simulink model "gm_soc_dvbs2_fpga"  (R2025b)
settings: Solver=VariableStepAuto  StartTime=0.0  StopTime=10.0  RelTol=1e-3
InitFcn:
  | soc_dvbs2_init;
undefined symbols (not defined in the file or in its folder): Add, coefficientsLog, coefficientsSqrt1, coefficientsSqrt2, dataBits, Deinterleaver, designMultirateFIR, noisePow, Shift, Short, soc_dvbs2_designFIRFilter, soc_dvbs2_txPacketBits, syncWord, txDataOut, txFiltCoeff, XData
libraries: simulink x304, hdlsllib x265, dspsigops x15, dsphdlfiltering2 x8, hdlmdlgenlib x6, dsphdlsigops2 x5, commseqgen3 x5, dsphdlmathfun2 x3, hwlogicconnlib x2, whdledac x2, commhdlcrc x2, whdlutilities x1
(part 3 of 36)

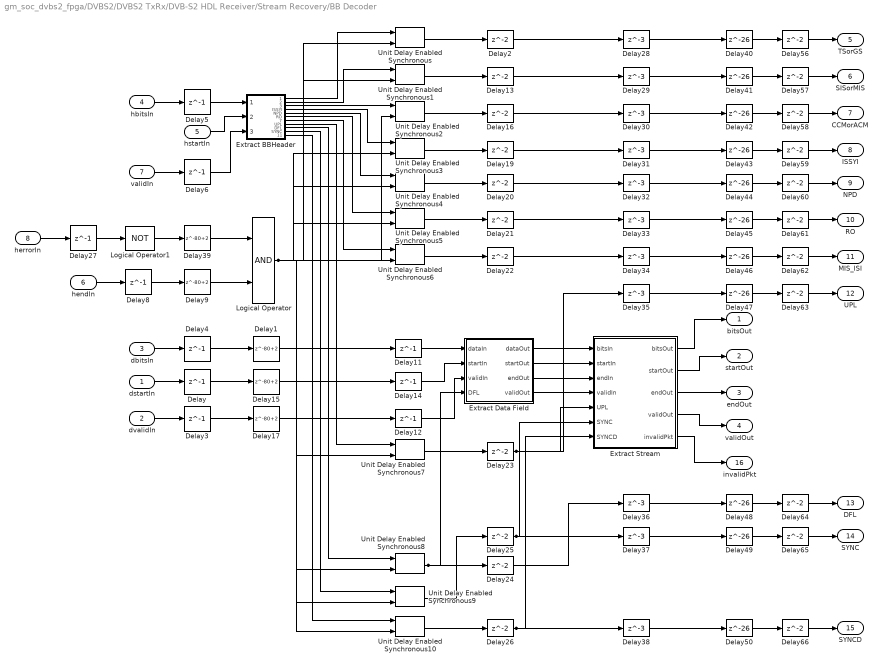
== system gm_soc_dvbs2_fpga/DVBS2/DVBS2 TxRx/DVB-S2 HDL Receiver/Stream Recovery/BB Decoder ==
  dstartIn : Inport  OutDataTypeStr=boolean  PortDimensions=1  SampleTime=7.8125e-09
  dvalidIn : Inport  Port=2  OutDataTypeStr=boolean  PortDimensions=1  SampleTime=7.8125e-09
  dbitsIn : Inport  Port=3  OutDataTypeStr=boolean  PortDimensions=1  SampleTime=7.8125e-09
  hbitsIn : Inport  Port=4  OutDataTypeStr=boolean  PortDimensions=1  SampleTime=7.8125e-09
  hstartIn : Inport  Port=5  OutDataTypeStr=boolean  PortDimensions=1  SampleTime=7.8125e-09
  hendIn : Inport  Port=6  OutDataTypeStr=boolean  PortDimensions=1  SampleTime=7.8125e-09
  validIn : Inport  Port=7  OutDataTypeStr=boolean  PortDimensions=1  SampleTime=7.8125e-09
  herrorIn : Inport  Port=8  OutDataTypeStr=boolean  PortDimensions=1  SampleTime=7.8125e-09
  Delay{,3..6,8,11..12,14,27} (10 alike) : Delay  DelayLength=1
  Delay{1,9,15,17,39} (5 alike) : Delay  DelayLength=80+2
  Delay{2,13,16,19..26,56..66} (22 alike) : Delay
  Delay{28..38} (11 alike) : Delay  DelayLength=3
  Delay{40..50} (11 alike) : Delay  DelayLength=26
  Extract BBHeader : Subsystem
      mask init:
      | ii = double(5);
  Extract Data Field : Subsystem
  Extract Stream : Subsystem
  Logical Operator : Logic  AllPortsSameDT=off  OutDataTypeStr=boolean
  Logical Operator1 : Logic  Operator=NOT  AllPortsSameDT=off  OutDataTypeStr=boolean
  Unit Delay Enabled Synchronous{,1..10} (11 alike) : hdlsllib/Discrete/Unit Delay Enabled Synchronous  InitialCondition=0.0  SampleTime=-1
  bitsOut : Outport  SampleTime=7.8125e-09
  startOut : Outport  Port=2  SampleTime=7.8125e-09
  endOut : Outport  Port=3  SampleTime=7.8125e-09
  validOut : Outport  Port=4  SampleTime=7.8125e-09
  TSorGS : Outport  Port=5  SampleTime=7.8125e-09
  SISorMIS : Outport  Port=6  SampleTime=7.8125e-09
  CCMorACM : Outport  Port=7  SampleTime=7.8125e-09
  ISSYI : Outport  Port=8  SampleTime=7.8125e-09
  NPD : Outport  Port=9  SampleTime=7.8125e-09
  RO : Outport  Port=10  SampleTime=7.8125e-09
  MIS_ISI : Outport  Port=11  SampleTime=7.8125e-09
  UPL : Outport  Port=12  SampleTime=7.8125e-09
  DFL : Outport  Port=13  SampleTime=7.8125e-09
  SYNC : Outport  Port=14  SampleTime=7.8125e-09
  SYNCD : Outport  Port=15  SampleTime=7.8125e-09
  invalidPkt : Outport  Port=16  SampleTime=7.8125e-09
  wires:
  Delay27/1 -> Logical Operator1/1
  herrorIn/1 -> Delay27/1
  Unit Delay Enabled Synchronous/1 -> Delay2/1
  Delay17/1 -> Delay12/1
  hbitsIn/1 -> Delay5/1
  Delay2/1 -> Delay28/1
  hendIn/1 -> Delay8/1
  validIn/1 -> Delay6/1
  Logical Operator1/1 -> Delay39/1
  Delay8/1 -> Delay9/1
  dbitsIn/1 -> Delay4/1
  Delay16/1 -> Delay30/1
  Unit Delay Enabled Synchronous7/1 -> Delay23/1
  dstartIn/1 -> Delay/1
  Delay23/1 -> Delay35/1, Extract Stream/5(UPL)
  dvalidIn/1 -> Delay3/1
  Delay5/1 -> Extract BBHeader/1(bitsIn)
  Delay20/1 -> Delay32/1
  Delay12/1 -> Extract Data Field/3(validIn)
  hstartIn/1 -> Extract BBHeader/2(reset)
  Delay6/1 -> Extract BBHeader/3(validIn)
  Delay39/1 -> Logical Operator/1
  Delay9/1 -> Logical Operator/2
  Delay4/1 -> Delay1/1
  Unit Delay Enabled Synchronous8/1 -> Delay24/1, Extract Data Field/4(DFL)
  Delay/1 -> Delay15/1
  Extract BBHeader/1(TSorGS) -> Unit Delay Enabled Synchronous/1
  Extract Stream/5(invalidPkt) -> invalidPkt/1
  Delay3/1 -> Delay17/1
  Extract BBHeader/2(SISorMIS) -> Unit Delay Enabled Synchronous1/1
  Extract Data Field/3(endOut) -> Extract Stream/3(endIn)
  Extract BBHeader/3(CCMorACM) -> Unit Delay Enabled Synchronous2/1
  Extract BBHeader/4(ISSYI) -> Unit Delay Enabled Synchronous3/1
  Extract BBHeader/5(NPD) -> Unit Delay Enabled Synchronous4/1
  Extract BBHeader/6(RO) -> Unit Delay Enabled Synchronous5/1
  Unit Delay Enabled Synchronous3/1 -> Delay19/1
  Extract BBHeader/7(MIS_ISI) -> Unit Delay Enabled Synchronous6/1
  Extract BBHeader/8(UPL) -> Unit Delay Enabled Synchronous7/1
  Extract Data Field/4(validOut) -> Extract Stream/4(validIn)
  Extract BBHeader/9(DFL) -> Unit Delay Enabled Synchronous8/1
  Delay29/1 -> Delay41/1
  Extract BBHeader/10(SYNC) -> Unit Delay Enabled Synchronous9/1
  Extract Data Field/2(startOut) -> Extract Stream/2(startIn)
  Extract BBHeader/11(SYNCD) -> Unit Delay Enabled Synchronous10/1
  Logical Operator/1 -> Unit Delay Enabled Synchronous9/2, Unit Delay Enabled Synchronous7/2, Unit Delay Enabled Synchronous8/2, Unit Delay Enabled Synchronous4/2, Unit Delay Enabled Synchronous3/2, Unit Delay Enabled Synchronous6/2, Unit Delay Enabled Synchronous2/2, Unit Delay Enabled Synchronous10/2, Unit Delay Enabled Synchronous5/2, Unit Delay Enabled Synchronous1/2, Unit Delay Enabled Synchronous/2
  Delay19/1 -> Delay31/1
  Delay1/1 -> Delay11/1
  Delay15/1 -> Delay14/1
  Delay24/1 -> Delay36/1
  Unit Delay Enabled Synchronous1/1 -> Delay13/1
  Unit Delay Enabled Synchronous2/1 -> Delay16/1
  Extract Data Field/1(dataOut) -> Extract Stream/1(bitsIn)
  Unit Delay Enabled Synchronous4/1 -> Delay20/1
  Unit Delay Enabled Synchronous5/1 -> Delay21/1
  Delay66/1 -> SYNCD/1
  Unit Delay Enabled Synchronous6/1 -> Delay22/1
  Delay11/1 -> Extract Data Field/1(dataIn)
  Delay22/1 -> Delay34/1
  Delay14/1 -> Extract Data Field/2(startIn)
  Unit Delay Enabled Synchronous9/1 -> Delay25/1
  Unit Delay Enabled Synchronous10/1 -> Delay26/1
  Delay21/1 -> Delay33/1
  Delay13/1 -> Delay29/1
  Delay25/1 -> Delay37/1, Extract Stream/6(SYNC)
  Delay26/1 -> Delay38/1, Extract Stream/7(SYNCD)
  Delay28/1 -> Delay40/1
  Delay30/1 -> Delay42/1
  Delay31/1 -> Delay43/1
  Delay32/1 -> Delay44/1
  Delay33/1 -> Delay45/1
  Delay34/1 -> Delay46/1
  Delay35/1 -> Delay47/1
  Extract Stream/1(bitsOut) -> bitsOut/1
  Extract Stream/2(startOut) -> startOut/1
  Extract Stream/3(endOut) -> endOut/1
  Extract Stream/4(validOut) -> validOut/1
  Delay36/1 -> Delay48/1
  Delay37/1 -> Delay49/1
  Delay38/1 -> Delay50/1
  Delay40/1 -> Delay56/1
  Delay41/1 -> Delay57/1
  Delay42/1 -> Delay58/1
  Delay43/1 -> Delay59/1
  Delay44/1 -> Delay60/1
  Delay45/1 -> Delay61/1
  Delay46/1 -> Delay62/1
  Delay47/1 -> Delay63/1
  Delay48/1 -> Delay64/1
  Delay49/1 -> Delay65/1
  Delay50/1 -> Delay66/1
  Delay56/1 -> TSorGS/1
  Delay57/1 -> SISorMIS/1
  Delay58/1 -> CCMorACM/1
  Delay59/1 -> ISSYI/1
  Delay60/1 -> NPD/1
  Delay61/1 -> RO/1
  Delay62/1 -> MIS_ISI/1
  Delay63/1 -> UPL/1
  Delay64/1 -> DFL/1
  Delay65/1 -> SYNC/1

== system gm_soc_dvbs2_fpga/DVBS2/DVBS2 TxRx/DVB-S2 HDL Receiver/Stream Recovery/BB Demultiplexer ==
  bitsIn : Inport  OutDataTypeStr=boolean  PortDimensions=1  SampleTime=7.8125e-09
  startIn : Inport  Port=2  OutDataTypeStr=boolean  PortDimensions=1  SampleTime=7.8125e-09
  validIn : Inport  Port=3  OutDataTypeStr=boolean  PortDimensions=1  SampleTime=7.8125e-09
  Compare To Constant : simulink/Logic and Bit Operations/Compare To Constant  relop=<=  const=80 - 1  OutDataTypeStr=boolean
  Compare To Constant1 : simulink/Logic and Bit Operations/Compare To Constant  relop===  const=80 - 1  OutDataTypeStr=boolean
  Compare To Constant2 : simulink/Logic and Bit Operations/Compare To Constant  relop===  const=80  OutDataTypeStr=boolean
  Delay1 : Delay  DelayLength=1
  Delay2 : Delay  DelayLength=1
  Delay3 : Delay  DelayLength=1
  HDL Counter : hdlsllib/Sources/HDL Counter  CountType=Free running  CountInit=0  CountStep=1  CountMax=25  CountFromType=Initial value  CountFrom=0  CountResetPort=on  CountLoadPort=off  CountEnbPort=on  CountDirPort=off  CountHitOutputPort=off  CountDataType=Unsigned  CountWordLen=nextpow2(58192)  CountFracLen=0  CountSampTime=-1
  Logical Operator{,1,3..4} (4 alike) : Logic  AllPortsSameDT=off  OutDataTypeStr=boolean
  Logical Operator2 : Logic  Operator=NOT  AllPortsSameDT=off  OutDataTypeStr=boolean
  dstartOut : Outport  SampleTime=7.8125e-09
  dValidOut : Outport  Port=2  SampleTime=7.8125e-09
  bitsOut : Outport  Port=3  SampleTime=7.8125e-09
  hstartOut : Outport  Port=4  SampleTime=7.8125e-09
  hendOut : Outport  Port=5  SampleTime=7.8125e-09
  hvalidOut : Outport  Port=6  SampleTime=7.8125e-09
  wires:
  Compare To Constant1/1 -> Logical Operator1/1
  Delay1/1 -> hstartOut/1
  Compare To Constant2/1 -> Logical Operator4/1
  Logical Operator3/1 -> dValidOut/1
  Delay3/1 -> Logical Operator4/2, Logical Operator3/2, Logical Operator/2, HDL Counter/2, Logical Operator1/2
  Logical Operator4/1 -> dstartOut/1
  validIn/1 -> Delay3/1
  bitsIn/1 -> Delay2/1
  startIn/1 -> Delay1/1, HDL Counter/1
  Logical Operator1/1 -> hendOut/1
  Delay2/1 -> bitsOut/1
  HDL Counter/1 -> Compare To Constant2/1, Compare To Constant1/1, Compare To Constant/1
  Compare To Constant/1 -> Logical Operator2/1, Logical Operator/1
  Logical Operator2/1 -> Logical Operator3/1
  Logical Operator/1 -> hvalidOut/1

== system gm_soc_dvbs2_fpga/DVBS2/DVBS2 TxRx/DVB-S2 HDL Receiver/Stream Recovery/BB Descrambler ==
  bitsIn : Inport  OutDataTypeStr=boolean  PortDimensions=1  SampleTime=7.8125e-09
  startIn : Inport  Port=2  OutDataTypeStr=boolean  PortDimensions=1  SampleTime=7.8125e-09
  validIn : Inport  Port=3  OutDataTypeStr=boolean  PortDimensions=1  SampleTime=7.8125e-09
  Data Type Conversion : DataTypeConversion  OutDataTypeStr=boolean  SaturateOnIntegerOverflow=off  RndMeth=Floor
  Logical Operator : Logic  Operator=XOR  AllPortsSameDT=off  OutDataTypeStr=boolean
  Subsystem : Subsystem
  bitsOut : Outport  SampleTime=7.8125e-09
  startOut : Outport  Port=2  SampleTime=7.8125e-09
  validOut : Outport  Port=3  SampleTime=7.8125e-09
  wires:
  startIn/1 -> Subsystem/1(In1), startOut/1
  bitsIn/1 -> Logical Operator/2
  validIn/1 -> Subsystem/Enable, validOut/1
  Logical Operator/1 -> bitsOut/1
  Data Type Conversion/1 -> Logical Operator/1
  Subsystem/1(Out1) -> Data Type Conversion/1

== system gm_soc_dvbs2_fpga/DVBS2/DVBS2 TxRx/DVB-S2 HDL Receiver/Stream Recovery/BB Header CRC Check ==
  dstartIn : Inport  OutDataTypeStr=boolean  PortDimensions=1  SampleTime=7.8125e-09
  dValidIn : Inport  Port=2  OutDataTypeStr=boolean  PortDimensions=1  SampleTime=7.8125e-09
  bitsIn : Inport  Port=3  OutDataTypeStr=boolean  PortDimensions=1  SampleTime=7.8125e-09
  hstartIn : Inport  Port=4  OutDataTypeStr=boolean  PortDimensions=1  SampleTime=7.8125e-09
  hendIn : Inport  Port=5  OutDataTypeStr=boolean  PortDimensions=1  SampleTime=7.8125e-09
  hvalidIn : Inport  Port=6  OutDataTypeStr=boolean  PortDimensions=1  SampleTime=7.8125e-09
  Delay{,1..3,8..13,15} (11 alike) : Delay  DelayLength=1
  Delay4 : Delay  DelayLength=26
  Delay6 : Delay  DelayLength=26
  Delay7 : Delay  DelayLength=26
  Discard CRC failed Frame : Subsystem
  General CRC Syndrome Detector HDL Optimized : commhdlcrc/General CRC Syndrome Detector HDL Optimized  Polynomial=[1 1 1 0 1 0 1 0 1]  InitialState=0  DirectMethod=off  ReflectInput=off  ReflectCRCChecksum=off  FinalXORValue=0  SimulateUsing=Code generation
  dstartOut : Outport  SampleTime=7.8125e-09
  dvalidIn : Outport  Port=2  SampleTime=7.8125e-09
  dbitsOut : Outport  Port=3  SampleTime=7.8125e-09
  hbitsOut : Outport  Port=4  SampleTime=7.8125e-09
  hstartOut : Outport  Port=5  SampleTime=7.8125e-09
  hendOut : Outport  Port=6  SampleTime=7.8125e-09
  hvalidOut : Outport  Port=7  SampleTime=7.8125e-09
  herrorOut : Outport  Port=8  SampleTime=7.8125e-09
  wires:
  General CRC Syndrome Detector HDL Optimized/1 -> Delay8/1
  dstartIn/1 -> Delay15/1
  dValidIn/1 -> Delay13/1
  bitsIn/1 -> Delay9/1
  hendIn/1 -> Delay11/1
  hvalidIn/1 -> Delay12/1
  hstartIn/1 -> Delay10/1
  Delay12/1 -> General CRC Syndrome Detector HDL Optimized/4
  Delay15/1 -> Delay4/1
  Delay13/1 -> Delay6/1
  Delay9/1 -> Delay7/1, General CRC Syndrome Detector HDL Optimized/1
  Delay8/1 -> hbitsOut/1
  Delay10/1 -> General CRC Syndrome Detector HDL Optimized/2
  Delay11/1 -> General CRC Syndrome Detector HDL Optimized/3
  Delay4/1 -> Discard CRC failed Frame/1(startIn)
  Delay6/1 -> Discard CRC failed Frame/2(validIn)
  Delay7/1 -> Discard CRC failed Frame/3(bitsIn)
  General CRC Syndrome Detector HDL Optimized/2 -> Delay3/1
  General CRC Syndrome Detector HDL Optimized/3 -> Delay2/1, Discard CRC failed Frame/5(errorValid)
  General CRC Syndrome Detector HDL Optimized/4 -> Delay1/1
  General CRC Syndrome Detector HDL Optimized/5 -> Discard CRC failed Frame/4(err), Delay/1
  Discard CRC failed Frame/1(startOut) -> dstartOut/1
  Discard CRC failed Frame/2(validOut) -> dvalidIn/1
  Discard CRC failed Frame/3(bitsOut) -> dbitsOut/1
  Delay3/1 -> hstartOut/1
  Delay2/1 -> hendOut/1
  Delay1/1 -> hvalidOut/1
  Delay/1 -> herrorOut/1

== system gm_soc_dvbs2_fpga/DVBS2/DVBS2 TxRx/DVB-S2 HDL Receiver/Synchronizer and PL Header Decoder/Enable MODCOD  ==
  modcod : Inport  OutDataTypeStr=fixdt(0, 5, 0)  PortDimensions=1  SampleTime=2.5e-07
  enb : Inport  Port=2  OutDataTypeStr=boolean  PortDimensions=1  SampleTime=2.5e-07
  Constant : Constant  Value=0  OutDataTypeStr=fixdt(0, 5, 0)  SampleTime=-1
  Constant1 : Constant  Value=modcodToZero  OutDataTypeStr=boolean  SampleTime=-1
  Switch : Switch  Criteria=u2 ~= 0  OutDataTypeStr=fixdt(0, 5, 0)  SaturateOnIntegerOverflow=off  InputSameDT=off
  Switch1 : Switch  Criteria=u2 ~= 0  OutDataTypeStr=fixdt(0, 5, 0)  SaturateOnIntegerOverflow=off  InputSameDT=off
  modcodOut : Outport  SampleTime=2.5e-07
  wires:
  Switch1/1 -> modcodOut/1
  Constant1/1 -> Switch1/2
  Constant/1 -> Switch/3
  enb/1 -> Switch/2
  Switch/1 -> Switch1/1
  modcod/1 -> Switch1/3, Switch/1

== system gm_soc_dvbs2_fpga/DVBS2/DVBS2 TxRx/DVB-S2 HDL Receiver/Synchronizer and PL Header Decoder/Fine Phase Synchronizer ==
  dataIn : Inport  OutDataTypeStr=fixdt(1, 18, 13)  PortDimensions=1  SampleTime=2.5e-07
      settings: SignalType=complex
  validIn : Inport  Port=2  OutDataTypeStr=boolean  PortDimensions=1  SampleTime=2.5e-07
  endOfPLSCIn : Inport  Port=3  OutDataTypeStr=boolean  PortDimensions=1  SampleTime=2.5e-07
  mod : Inport  Port=4  OutDataTypeStr=fixdt(0, 2, 0)  PortDimensions=1  SampleTime=2.5e-07
  En : Inport  Port=5  OutDataTypeStr=boolean  PortDimensions=1  SampleTime=2.5e-07
  rst : Inport  Port=6  OutDataTypeStr=boolean  PortDimensions=1  SampleTime=2.5e-07
  Data Type Conversion : DataTypeConversion  OutDataTypeStr=fixdt(1, 18, 14)  SampleTime=2.5e-07  SaturateOnIntegerOverflow=off  RndMeth=Floor
  Data Type Conversion1 : DataTypeConversion  OutDataTypeStr=fixdt(1, 22, 14)  SampleTime=2.5e-07  SaturateOnIntegerOverflow=off  RndMeth=Floor
  Delay{1..4,12..14} (7 alike) : Delay  DelayLength=double(1)  InitialCondition=0  SampleTime=2.5e-07
  Delay{5..11,15..16} (9 alike) : Delay  DelayLength=double(2)  InitialCondition=0  SampleTime=2.5e-07
  Direct Digital Synthesis : Subsystem
  Loop Filter : Subsystem
  Math Function : Math  Operator=conj  OutDataTypeStr=fixdt(1, 16, 14)
  Phase Error Detector : Subsystem
  Power Q and Beta Offset Rotation : Subsystem
  Product : Product  Inputs=**  OutDataTypeStr=fixdt(1, 34, 27)  SampleTime=2.5e-07
  dataOut : Outport  SampleTime=2.5e-07
  validOut : Outport  Port=2  SampleTime=2.5e-07
  endOfPLSC : Outport  Port=3  SampleTime=2.5e-07
  wires:
  validIn/1 -> Delay2/1
  endOfPLSCIn/1 -> Delay3/1
  dataIn/1 -> Delay4/1
  Phase Error Detector/1(e) -> Loop Filter/1(e)
  Product/1 -> Delay7/1
  Delay8/1 -> Delay10/1
  Delay4/1 -> Delay5/1
  Delay2/1 -> Delay8/1
  Delay5/1 -> Product/1
  Delay3/1 -> Delay9/1
  Delay7/1 -> Data Type Conversion1/1
  Delay9/1 -> Delay11/1
  Delay10/1 -> Delay13/1
  Delay11/1 -> Delay14/1
  Delay13/1 -> validOut/1
  Loop Filter/1(v) -> Direct Digital Synthesis/1(v)
  mod/1 -> Delay1/1
  Delay14/1 -> endOfPLSC/1
  Data Type Conversion/1 -> dataOut/1
  Data Type Conversion1/1 -> Delay12/1, Delay15/1
  En/1 -> Loop Filter/2(En)
  Delay1/1 -> Delay16/1
  Direct Digital Synthesis/1(xph) -> Math Function/1
  Delay12/1 -> Data Type Conversion/1
  Math Function/1 -> Delay6/1
  Delay15/1 -> Power Q and Beta Offset Rotation/1(dataIn)
  Delay16/1 -> Power Q and Beta Offset Rotation/2(mod)
  Power Q and Beta Offset Rotation/1(dataOut) -> Phase Error Detector/1(dataIn)
  rst/1 -> Loop Filter/3(rst)
  Loop Filter/2(rstOut) -> Direct Digital Synthesis/2(rst)
  Delay6/1 -> Product/2

== system gm_soc_dvbs2_fpga/DVBS2/DVBS2 TxRx/DVB-S2 HDL Receiver/Synchronizer and PL Header Decoder/PL Header Recovery ==
  dataIn : Inport  OutDataTypeStr=fixdt(1, 18, 13)  PortDimensions=1  SampleTime=2.5e-07
      settings: SignalType=complex
  validIn : Inport  Port=2  OutDataTypeStr=boolean  PortDimensions=1  SampleTime=2.5e-07
  endOfSOF : Inport  Port=3  OutDataTypeStr=boolean  PortDimensions=1  SampleTime=2.5e-07
  hasPilots : Inport  Port=4  OutDataTypeStr=boolean  PortDimensions=1  SampleTime=2.5e-07
  Bus Creator : BusCreator  Inputs=2
  Delay{,1..3,5,11..20} (15 alike) : Delay  DelayLength=1
  Delay10 : Delay  DelayLength=46
  Delay4 : Delay  DelayLength=3
  Delay6 : Delay  DelayLength=3
  Delay7 : Delay  DelayLength=3
  Delay8 : Delay  DelayLength=46
  Delay9 : Delay  DelayLength=46
  PL Frame Demultiplexer : Subsystem
  PL Header Decoder : Subsystem
  Unit Delay Enabled Synchronous : hdlsllib/Discrete/Unit Delay Enabled Synchronous  InitialCondition=0.0  SampleTime=-1
  Unit Delay Enabled Synchronous1 : hdlsllib/Discrete/Unit Delay Enabled Synchronous  InitialCondition=0.0  SampleTime=-1
  Unit Delay Enabled Synchronous2 : hdlsllib/Discrete/Unit Delay Enabled Synchronous  InitialCondition=0.0  SampleTime=-1
  PLSCDiag : Outport  VectorParamsAs1DForOutWhenUnconnected=off
  dataOut : Outport  Port=2  SampleTime=2.5e-07  VectorParamsAs1DForOutWhenUnconnected=off
  validOut : Outport  Port=3  SampleTime=2.5e-07  VectorParamsAs1DForOutWhenUnconnected=off
  endOfPLSC : Outport  Port=4  SampleTime=2.5e-07  VectorParamsAs1DForOutWhenUnconnected=off
  modcod : Outport  Port=5  SampleTime=2.5e-07  VectorParamsAs1DForOutWhenUnconnected=off
  FEC : Outport  Port=6  SampleTime=2.5e-07  VectorParamsAs1DForOutWhenUnconnected=off
  wires:
  endOfSOF/1 -> Delay2/1
  dataIn/1 -> Delay5/1
  validIn/1 -> Delay3/1
  PL Frame Demultiplexer/1(hValid) -> PL Header Decoder/4(validIn), Bus Creator/2  "PLSCSymbValid"
  hasPilots/1 -> Delay1/1
  Delay3/1 -> PL Frame Demultiplexer/2(validIn)
  Delay2/1 -> Delay7/1, PL Frame Demultiplexer/1(endOfSOFIn), Unit Delay Enabled Synchronous1/2
  Delay5/1 -> Delay4/1
  Delay1/1 -> Unit Delay Enabled Synchronous1/1
  Delay4/1 -> PL Header Decoder/1(dataIn), Bus Creator/1, Delay10/1  "PLSCSymb"
  Unit Delay Enabled Synchronous1/1 -> Delay6/1
  Delay7/1 -> PL Header Decoder/3(endOfSOF)
  PL Frame Demultiplexer/2(dValid) -> Delay8/1
  PL Frame Demultiplexer/3(endOfPLSC) -> Delay9/1
  Delay10/1 -> Delay12/1
  Bus Creator/1 -> PLSCDiag/1
  Delay6/1 -> PL Header Decoder/2(hasPilots)
  Delay8/1 -> Delay11/1
  Delay9/1 -> Delay/1
  Delay12/1 -> Delay13/1
  PL Header Decoder/1(modcod) -> Delay14/1
  Delay11/1 -> Delay17/1
  PL Header Decoder/2(FECFrame) -> Delay15/1
  Delay/1 -> Delay18/1
  Delay13/1 -> Delay16/1
  Delay14/1 -> Unit Delay Enabled Synchronous/1
  Delay17/1 -> Delay19/1
  Delay15/1 -> Unit Delay Enabled Synchronous2/1
  Delay18/1 -> Unit Delay Enabled Synchronous2/2, Unit Delay Enabled Synchronous/2, Delay20/1
  Delay16/1 -> dataOut/1
  Unit Delay Enabled Synchronous/1 -> modcod/1
  Delay19/1 -> validOut/1
  Unit Delay Enabled Synchronous2/1 -> FEC/1
  Delay20/1 -> endOfPLSC/1

== system gm_soc_dvbs2_fpga/DVBS2/DVBS2 TxRx/DVB-S2 HDL Receiver/Synchronizer and PL Header Decoder/Source Encoding ==
  modcod : Inport  OutDataTypeStr=fixdt(0, 5, 0)  PortDimensions=1  SampleTime=2.5e-07
  Delay1 : Delay  DelayLength=1
  Delay12 : Delay  DelayLength=1
  MATLAB Function : Subsystem
  MATLAB Function_term1 : Terminator
  mod : Outport  SampleTime=2.5e-07
  wires:
  MATLAB Function/2(isdummy) -> MATLAB Function_term1/1
  modcod/1 -> Delay12/1
  Delay12/1 -> MATLAB Function/1(In)
  MATLAB Function/1(out) -> Delay1/1
  Delay1/1 -> mod/1

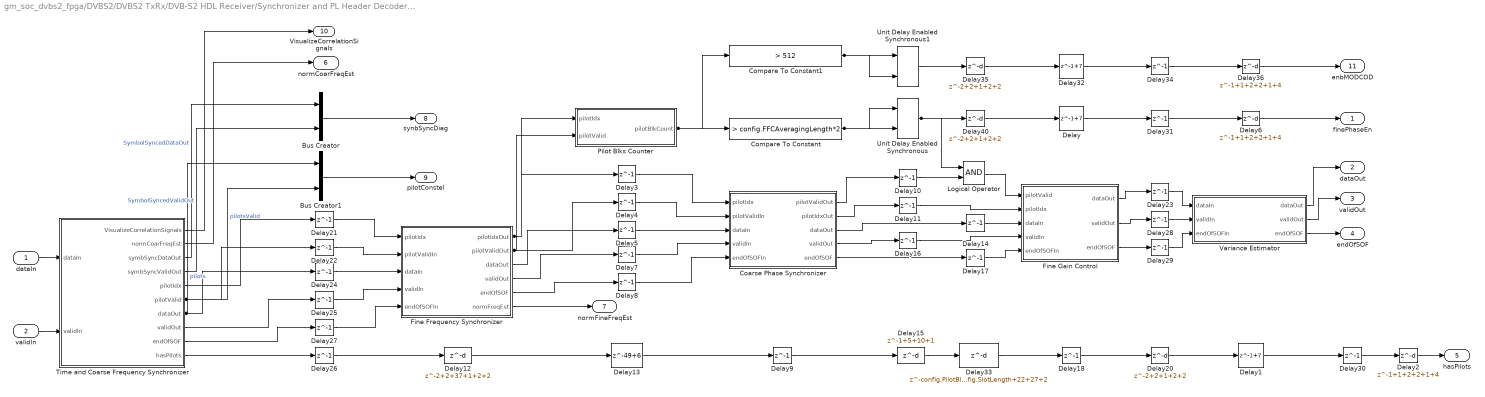
== system gm_soc_dvbs2_fpga/DVBS2/DVBS2 TxRx/DVB-S2 HDL Receiver/Synchronizer and PL Header Decoder/Time Frequency and Coarse Phase Synchronizer ==
  dataIn : Inport  OutDataTypeStr=fixdt(1, 18, 15)  PortDimensions=1  SampleTime=6.25e-08
      settings: SignalType=complex
  validIn : Inport  Port=2  OutDataTypeStr=boolean  PortDimensions=1  SampleTime=6.25e-08
  Bus Creator : BusCreator  Inputs=2
  Bus Creator1 : BusCreator  Inputs=2
  Coarse Phase Synchronizer : Subsystem
  Compare To Constant : simulink/Logic and Bit Operations/Compare To Constant  relop=>  const=config.FFCAveragingLength*2  OutDataTypeStr=boolean
  Compare To Constant1 : simulink/Logic and Bit Operations/Compare To Constant  relop=>  const=512  OutDataTypeStr=boolean
  Delay : Delay  DelayLength=1+7
  Delay1 : Delay  DelayLength=1+7
  Delay{3..5,7..11,14,16..18,21..31,34} (24 alike) : Delay  DelayLength=1
  Delay12 : Delay  DelayLength=2+2+37+1+2+2
  Delay13 : Delay  DelayLength=49+6
  Delay15 : Delay  DelayLength=1+5+10+1
  Delay2 : Delay  DelayLength=1+1+2+2+1+4
  Delay20 : Delay  DelayLength=2+2+1+2+2
  Delay32 : Delay  DelayLength=1+7
  Delay33 : Delay  DelayLength=config.PilotBlkFreq*config.SlotLength+22+27+2
  Delay35 : Delay  DelayLength=2+2+1+2+2
  Delay36 : Delay  DelayLength=1+1+2+2+1+4
  Delay40 : Delay  DelayLength=2+2+1+2+2
  Delay6 : Delay  DelayLength=1+1+2+2+1+4
  Fine Frequency Synchronizer : Subsystem
  Fine Gain Control : Subsystem
  Logical Operator : Logic  AllPortsSameDT=off  OutDataTypeStr=boolean
  Pilot Blks Counter : Subsystem
  Time and Coarse Frequency Synchronizer : Subsystem
  Unit Delay Enabled Synchronous : hdlsllib/Discrete/Unit Delay Enabled Synchronous  InitialCondition=0.0  SampleTime=-1
  Unit Delay Enabled Synchronous1 : hdlsllib/Discrete/Unit Delay Enabled Synchronous  InitialCondition=0.0  SampleTime=-1
  Variance Estimator : Subsystem
  finePhaseEn : Outport  SampleTime=2.5e-07
  dataOut : Outport  Port=2  SampleTime=2.5e-07
  validOut : Outport  Port=3  SampleTime=2.5e-07
  endOfSOF : Outport  Port=4  SampleTime=2.5e-07
  hasPilots : Outport  Port=5  SampleTime=2.5e-07
  normCoarFreqEst : Outport  Port=6  SampleTime=2.5e-07
  normFineFreqEst : Outport  Port=7  SampleTime=2.5e-07
  synbSyncDiag : Outport  Port=8
  pilotConstel : Outport  Port=9
  VisualizeCorrelationSignals : Outport  Port=10
  enbMODCOD : Outport  Port=11  SampleTime=2.5e-07
  wires:
  Delay24/1 -> Fine Frequency Synchronizer/3(dataIn)
  dataIn/1 -> Time and Coarse Frequency Synchronizer/1(dataIn)
  validIn/1 -> Time and Coarse Frequency Synchronizer/2(validIn)
  Delay/1 -> Delay31/1
  Time and Coarse Frequency Synchronizer/5(pilotIdx) -> Delay21/1
  Time and Coarse Frequency Synchronizer/3(symbSyncDataOut) -> Bus Creator/1  "SymbolSyncedDataOut"
  Time and Coarse Frequency Synchronizer/1(VisualizeCorrelationSignals) -> VisualizeCorrelationSignals/1
  Delay12/1 -> Delay13/1
  Time and Coarse Frequency Synchronizer/4(symbSyncValidOut) -> Bus Creator/2  "SymbolSyncedValidOut"
  Time and Coarse Frequency Synchronizer/2(normCoarFreqEst) -> normCoarFreqEst/1
  Time and Coarse Frequency Synchronizer/6(pilotValid) -> Bus Creator1/2, Delay22/1  "pilotsValid"
  Time and Coarse Frequency Synchronizer/7(dataOut) -> Bus Creator1/1, Delay24/1  "pilots"
  Time and Coarse Frequency Synchronizer/8(validOut) -> Delay25/1
  Unit Delay Enabled Synchronous/1 -> Logical Operator/1, Delay40/1
  Pilot Blks Counter/1(pilotBlkCount) -> Compare To Constant1/1, Compare To Constant/1
  Time and Coarse Frequency Synchronizer/9(endOfSOF) -> Delay27/1
  Fine Frequency Synchronizer/2(pilotValidOut) -> Delay4/1, Pilot Blks Counter/2(pilotValid)
  Time and Coarse Frequency Synchronizer/10(hasPilots) -> Delay26/1
  Bus Creator/1 -> synbSyncDiag/1
  Fine Frequency Synchronizer/5(endOfSOF) -> Delay8/1
  Bus Creator1/1 -> pilotConstel/1
  Delay21/1 -> Fine Frequency Synchronizer/1(pilotIdx)
  Delay22/1 -> Fine Frequency Synchronizer/2(pilotValidIn)
  Delay25/1 -> Fine Frequency Synchronizer/4(validIn)
  Delay27/1 -> Fine Frequency Synchronizer/5(endOfSOFIn)
  Delay26/1 -> Delay12/1
  Fine Frequency Synchronizer/1(pilotIdxOut) -> Delay3/1, Pilot Blks Counter/1(pilotIdx)
  Fine Frequency Synchronizer/3(dataOut) -> Delay5/1
  Fine Frequency Synchronizer/4(validOut) -> Delay7/1
  Fine Frequency Synchronizer/6(normFreqEst) -> normFineFreqEst/1
  Delay3/1 -> Coarse Phase Synchronizer/1(pilotIdx)
  Delay4/1 -> Coarse Phase Synchronizer/2(pilotValidIn)
  Coarse Phase Synchronizer/4(validOut) -> Delay16/1
  Variance Estimator/1(dataOut) -> dataOut/1
  Delay5/1 -> Coarse Phase Synchronizer/3(dataIn)
  Coarse Phase Synchronizer/2(pilotIdxOut) -> Delay11/1
  Delay7/1 -> Coarse Phase Synchronizer/4(validIn)
  Coarse Phase Synchronizer/1(pilotValidOut) -> Delay10/1
  Delay8/1 -> Coarse Phase Synchronizer/5(endOfSOFIn)
  Delay13/1 -> Delay9/1
  Compare To Constant/1 -> Unit Delay Enabled Synchronous/2, Unit Delay Enabled Synchronous/1
  Compare To Constant1/1 -> Unit Delay Enabled Synchronous1/2, Unit Delay Enabled Synchronous1/1
  Coarse Phase Synchronizer/3(dataOut) -> Delay14/1
  Coarse Phase Synchronizer/5(endOfSOF) -> Delay17/1
  Delay40/1 -> Delay/1
  Delay28/1 -> Variance Estimator/2(validIn)
  Delay9/1 -> Delay15/1
  Fine Gain Control/1(dataOut) -> Delay23/1
  Unit Delay Enabled Synchronous1/1 -> Delay35/1
  Delay10/1 -> Logical Operator/2
  Delay11/1 -> Fine Gain Control/2(pilotIdx)
  Delay16/1 -> Fine Gain Control/4(validIn)
  Delay14/1 -> Fine Gain Control/3(dataIn)
  Delay15/1 -> Delay33/1
  Delay35/1 -> Delay32/1
  Logical Operator/1 -> Fine Gain Control/1(pilotValid)
  Delay17/1 -> Fine Gain Control/5(endOfSOFIn)
  Delay33/1 -> Delay18/1
  Delay32/1 -> Delay34/1
  Fine Gain Control/2(validOut) -> Delay28/1
  Fine Gain Control/3(endOfSOF) -> Delay29/1
  Delay18/1 -> Delay20/1
  Delay34/1 -> Delay36/1
  Delay31/1 -> Delay6/1
  Delay23/1 -> Variance Estimator/1(dataIn)
  Delay29/1 -> Variance Estimator/3(endOfSOFIn)
  Delay20/1 -> Delay1/1
  Delay36/1 -> enbMODCOD/1
  Delay6/1 -> finePhaseEn/1
  Variance Estimator/2(validOut) -> validOut/1
  Variance Estimator/3(endOfSOF) -> endOfSOF/1
  Delay1/1 -> Delay30/1
  Delay30/1 -> Delay2/1
  Delay2/1 -> hasPilots/1
